simulink model "saturn_ib_stack_test"  (Simulink 6.2)
settings: Solver=ode4  SolverMode=SingleTasking  StartTime=-20.0  StopTime=620  FixedStep=0.005  RelTol=1e-3
values from neighbouring files (symbols this model uses):
  A_z_deg = 82.8200    (= 82.82)    [AS205_presettings.m]
  BN_1_sec = 14.4    [AS205_presettings.m]
  DeltaV_b_mps = 7.2381    [AS205_presettings.m]
  epsilon_2_sec = 15.0    (= 15)    [AS205_presettings.m]
  epsilon_prime_sec = 3.0    (= 3)    [AS205_presettings.m]
  i_deg = 28.89597    [AS205_presettings.m]
  lambda_0_deg = 102.32900    (= 102.329)    [AS205_presettings.m]
  lambda_L_deg = -80.561141    [AS205_presettings.m]
  pad_roll_L_deg = 100.0    (= 100)    [AS205_presettings.m]
  phi_L_deg = 28.521963    [AS205_presettings.m]
  phi_L_prime_deg = 28.360795    [AS205_presettings.m]
  R_L_m = 6373385.0    (= 6373385)    [AS205_presettings.m]
  R_T_m = 6570774.0    (= 6570774)    [AS205_presettings.m]
  T3_FM_sec = 6.08    [AS205_presettings.m]
  T_HSL_sec = 5.0    (= 5)    [AS205_presettings.m]
  Theta_T_deg = 0.000    (= 0)    [AS205_presettings.m]
  V_T_mps = 7780.976    [AS205_presettings.m]
  Xdotdot_VGT_mps2 = -9.251    [AS205_presettings.m]
undefined symbols (not defined in the file or in its folder): e0_0, e1_0, e2_0, e3_0, m, s
libraries: simulink x99, aerolibconvert x83, aerolibutil x63, aerolibtransform2 x34, aerolibasang x2, aerolibatmos2 x2, aerolib6dofsys x2
(part 4 of 7)

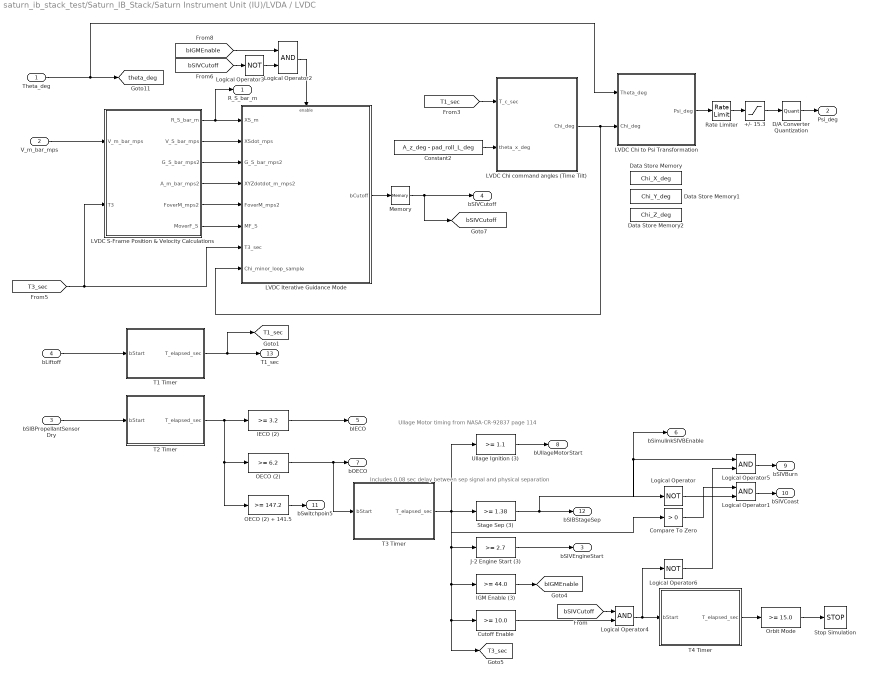
== system saturn_ib_stack_test/Saturn_IB_Stack/Saturn Instrument Unit (IU)/LVDA / LVDC ==
  note: Includes 0.08 sec delay between sep signal
      | and physical separation
  note: Ullage Motor timing
      | from NASA-CR-92837 page 114
  Theta_deg : Inport  Port=1  LatchInput=off
  V_m_bar_mps : Inport  Port=2  LatchInput=off
  bSIBPropellantSensorDry : Inport  Port=3  LatchInput=off
  bLiftoff : Inport  Port=4  PortDimensions=1  DataType=boolean  LatchInput=off
  +/- 15.3 : Saturate  UpperLimit=15.3  LowerLimit=-15.3
  Compare To Zero : simulink/Logic and Bit Operations/Compare To Zero  relop=>  LogicOutDataTypeMode=uint8  ZeroCross=off
  Constant2 : Constant  Value=A_z_deg - pad_roll_L_deg
  Cutoff Enable : simulink/Logic and Bit Operations/Compare To Constant  relop=>=  const=10.0  LogicOutDataTypeMode=boolean  ZeroCross=off
  D/A Converter Quantization : Quantizer  QuantizationInterval=0.0575
  Data Store Memory : DataStoreMemory  DataStoreName=Chi_X_deg  InitialValue=A_z_deg - pad_roll_L_deg  DataType=double
  Data Store Memory1 : DataStoreMemory  DataStoreName=Chi_Y_deg  InitialValue=0  DataType=double
  Data Store Memory2 : DataStoreMemory  DataStoreName=Chi_Z_deg  InitialValue=0  DataType=double
  IECO (2) : simulink/Logic and Bit Operations/Compare To Constant  relop=>=  const=3.2  LogicOutDataTypeMode=boolean  ZeroCross=off
  IGM Enable (3) : simulink/Logic and Bit Operations/Compare To Constant  relop=>=  const=44.0  LogicOutDataTypeMode=boolean  ZeroCross=off
  J-2 Engine Start (3) : simulink/Logic and Bit Operations/Compare To Constant  relop=>=  const=2.7  LogicOutDataTypeMode=boolean  ZeroCross=off
  LVDC Chi command angles (Time Tilt) : Subsystem
  LVDC Chi to Psi Transformation : Subsystem
  LVDC Iterative Guidance Mode : Subsystem  mask{lambda_dot_deg_per_sec=0.0, AP_dcm=[-0.18749569 -0.98223810 -0.73231298; 0.98202016 -0.18761026 0.20946740; -0.21948577 -0.32640360 0.99975374], T10_sec=286.9, A0_sec=458.9, A1=-1.194, Tr1=1.8, Tr2=0.0, Tr3=0.0, T2_sec=0.0, delta_T_sec=1.6, tau_1_i_preset_sec=286.9, tau_3_i_preset_sec=116.0, tau_3_preset_sec=262.52, V_ex1_mps=4135.6997, V_ex3_mps=4192.6960, PC0_sec=60.0, tau_1_0_sec=528.0, C_0_sec=35.0, Mdot_1_kg_per_sec=243.687, Mdot_3_kg_per_sec=204.129}
      mask prompts: lambda_dot_deg_per_sec "lambda_dot (deg/sec)"; AP_dcm "AP"; T10_sec "T_10 (sec)"; A0_sec "A0 (sec)"; T2_sec "T2 (sec)"; tau_1_i_preset_sec "T_1_i  preset (sec)"; tau_3_i_preset_sec "T_3_i preset (sec)"; tau_3_preset_sec "tau_3 preset (sec)"; V_ex1_mps "V_ex1 (m/sec)"; V_ex3_mps "V_ex3 (m/sec)"; PC0_sec "PC0 (sec)"; tau_1_0_sec "T_1_0 (sec)"; C_0_sec "C_0 (sec)"; Mdot_1_kg_per_sec "Mdot_1 (kg/sec)"; Mdot_3_kg_per_sec "Mdot_3 (kg/sec)"
      settings: PermitHierarchicalResolution=ParametersOnly
  LVDC S-Frame Position & Velocity Calculations : Subsystem  mask{delta_T_sec=1.6}
      mask prompts: delta_T_sec "Major Loop Time Interval (sec)"
  Logical Operator : Logic  Operator=NOT  AllPortsSameDT=off  OutDataTypeMode=Boolean
  Logical Operator{1..2,4..5} (4 alike) : Logic  AllPortsSameDT=off  OutDataTypeMode=Boolean
  Logical Operator3 : Logic  Operator=NOT  AllPortsSameDT=off  OutDataTypeMode=Boolean
  Logical Operator6 : Logic  Operator=NOT  AllPortsSameDT=off  OutDataTypeMode=Boolean
  Memory : Memory  InheritSampleTime=on
  OECO (2) : simulink/Logic and Bit Operations/Compare To Constant  relop=>=  const=6.2  LogicOutDataTypeMode=boolean  ZeroCross=off
  OECO (2) + 141.5 : simulink/Logic and Bit Operations/Compare To Constant  relop=>=  const=147.2  LogicOutDataTypeMode=boolean  ZeroCross=off
  Orbit Mode : simulink/Logic and Bit Operations/Compare To Constant  relop=>=  const=15.0  LogicOutDataTypeMode=boolean  ZeroCross=off
  Rate Limiter : RateLimiter  RisingSlewLimit=12.0  FallingSlewLimit=-12.0  SampleTimeMode=inherited
  Stage Sep (3) : simulink/Logic and Bit Operations/Compare To Constant  relop=>=  const=1.38  LogicOutDataTypeMode=boolean  ZeroCross=off
  Stop Simulation : Stop
  T1 Timer : Subsystem
  T2 Timer : Subsystem
  T3 Timer : Subsystem
  T4 Timer : Subsystem
  Ullage Ignition (3) : simulink/Logic and Bit Operations/Compare To Constant  relop=>=  const=1.1  LogicOutDataTypeMode=boolean  ZeroCross=off
  R_S_bar_m : Outport
  Psi_deg : Outport  Port=2
  bSIVEngineStart : Outport  Port=3
  bSIVCutoff : Outport  Port=4
  bIECO : Outport  Port=5
  bSimulinkSIVBEnable : Outport  Port=6
  bOECO : Outport  Port=7
  bUllageMotorStart : Outport  Port=8
  bSIVBurn : Outport  Port=9
  bSIVCoast : Outport  Port=10
  bSwitchpoin5 : Outport  Port=11
  bSIBStageSep : Outport  Port=12
  T1_sec : Outport  Port=13
  tag scope: T1_sec=global, T3_sec=global, bIGMEnable=global, bSIVCutoff=global, theta_deg=global
  wires:
  Constant2/1 -> LVDC Chi command angles (Time Tilt)/2(theta_x_deg)
  +/- 15.3/1 -> D/A Converter Quantization/1
  LVDC Chi to Psi Transformation/1(Psi_deg) -> Rate Limiter/1
  Theta_deg/1 -> LVDC Chi to Psi Transformation/1(Theta_deg), [theta_deg]
  [T1_sec] -> LVDC Chi command angles (Time Tilt)/1(T_c_sec)
  T2 Timer/1(T_elapsed_sec) -> IECO (2)/1, OECO (2)/1, OECO (2) + 141.5/1
  OECO (2)/1 -> T3 Timer/1(bStart), bOECO/1
  T3 Timer/1(T_elapsed_sec) -> Stage Sep (3)/1, Ullage Ignition (3)/1, Compare To Zero/1, J-2 Engine Start (3)/1, IGM Enable (3)/1, [T3_sec], Cutoff Enable/1
  Stage Sep (3)/1 -> bSimulinkSIVBEnable/1, Logical Operator/1, Logical Operator5/1, bSIBStageSep/1
  bLiftoff/1 -> T1 Timer/1(bStart)
  T1 Timer/1(T_elapsed_sec) -> [T1_sec], T1_sec/1
  Logical Operator/1 -> Logical Operator1/2
  Compare To Zero/1 -> Logical Operator1/1
  LVDC S-Frame Position & Velocity Calculations/2(V_S_bar_mps) -> LVDC Iterative Guidance Mode/2(XSdot_mps)
  LVDC S-Frame Position & Velocity Calculations/1(R_S_bar_m) -> R_S_bar_m/1, LVDC Iterative Guidance Mode/1(XS_m)
  LVDC S-Frame Position & Velocity Calculations/3(G_S_bar_mps2) -> LVDC Iterative Guidance Mode/3(G_S_bar_mps2)
  IGM Enable (3)/1 -> [bIGMEnable]
  LVDC S-Frame Position & Velocity Calculations/5(FoverM_mps2) -> LVDC Iterative Guidance Mode/5(FoverM_mps2)
  LVDC S-Frame Position & Velocity Calculations/4(A_m_bar_mps2) -> LVDC Iterative Guidance Mode/4(XYZdotdot_m_mps2)
  LVDC Chi command angles (Time Tilt)/1(Chi_deg) -> LVDC Chi to Psi Transformation/2(Chi_deg), LVDC Iterative Guidance Mode/8(Chi_minor_loop_sample)
  [T3_sec] -> LVDC Iterative Guidance Mode/7(T3_sec), LVDC S-Frame Position & Velocity Calculations/2(T3)
  LVDC S-Frame Position & Velocity Calculations/6(MoverF_S) -> LVDC Iterative Guidance Mode/6(MF_S)
  Rate Limiter/1 -> +/- 15.3/1
  LVDC Iterative Guidance Mode/1(bCutoff) -> Memory/1
  Logical Operator3/1 -> Logical Operator2/2
  [bSIVCutoff] -> Logical Operator3/1
  [bIGMEnable] -> Logical Operator2/1
  Logical Operator2/1 -> LVDC Iterative Guidance Mode/Enable
  V_m_bar_mps/1 -> LVDC S-Frame Position & Velocity Calculations/1(V_m_bar_mps)
  D/A Converter Quantization/1 -> Psi_deg/1
  Memory/1 -> bSIVCutoff/1, [bSIVCutoff]
  IECO (2)/1 -> bIECO/1
  bSIBPropellantSensorDry/1 -> T2 Timer/1(bStart)
  Ullage Ignition (3)/1 -> bUllageMotorStart/1
  OECO (2) + 141.5/1 -> bSwitchpoin5/1
  Logical Operator1/1 -> bSIVCoast/1
  J-2 Engine Start (3)/1 -> bSIVEngineStart/1
  T4 Timer/1(T_elapsed_sec) -> Orbit Mode/1
  Orbit Mode/1 -> Stop Simulation/1
  [bSIVCutoff] -> Logical Operator4/1
  Logical Operator4/1 -> T4 Timer/1(bStart), Logical Operator6/1
  Cutoff Enable/1 -> Logical Operator4/2
  Logical Operator5/1 -> bSIVBurn/1
  Logical Operator6/1 -> Logical Operator5/2

== system saturn_ib_stack_test/Saturn_IB_Stack/Saturn Instrument Unit (IU)/ST-124M Stabilized Platform ==
  note: ECI orientation of the ST-124M
      | platform at Ground Reference
      | Release time
  note: ECI Orientation of the L/V
  q_ECI : Inport  Port=1  LatchInput=off
  ST124M DCM : Inport  Port=2  LatchInput=off
  A_b_mps2 : Inport  Port=3  PortDimensions=3  LatchInput=off
  +/- 45.0 deg : Saturate  UpperLimit=pi/4.0  LowerLimit=-pi/4.0
  Accelerometer Quantization : Quantizer  QuantizationInterval=0.05
  Angle Conversion8 : aerolibconvert/Angle Conversion  IU=rad  OU=deg
  Body to ECI : Product  Multiplication=Matrix(*)  RndMeth=Zero
  Demux5 : Demux  Outputs=3
  ECI to Platform : Product  Multiplication=Matrix(*)  RndMeth=Zero
  Fine Resolver Quantization : Quantizer  QuantizationInterval=0.00279
  Integrating Accelerometers : Integrator
  Math Function : Math  Operator=transpose  SaturateOnIntegerOverflow=on
  Math Function1 : Math  Operator=transpose  SaturateOnIntegerOverflow=on
  Math Function2 : Math  Operator=transpose  SaturateOnIntegerOverflow=on
  Memory : Memory  X0=[A_z_deg - pad_roll_L_deg 0.0 0.0]  InheritSampleTime=on
  Mux : Mux  Inputs=3
  Platform Gimbal Angles : Subsystem  AncestorBlock=aerolibtransform2/Direction Cosine Matrix to Euler Angles
      mask Type: DCM2Euler
      mask Description: Determine equivalent ST-124M Gimbal angles from the 3-by-3 direction cosine matrix (DCM). The input DCM transforms vectors from Body frame to S-Frame.  EDD Equation 2.3.3 was used to determine the correct Euler angle rotation sequence used in the ST-124M.
      mask Display: disp('DCM2Gimbal')
  Product9 : Product  Multiplication=Matrix(*)  RndMeth=Zero
  Quaternions to  Direction Cosine Matrix1 : aerolibtransform2/Quaternions to  Direction Cosine Matrix
  Gimbal Angles (deg) : Outport
  accumulated velocity (m/sec) : Outport  Port=2  DataType=double
  wires:
  q_ECI/1 -> Quaternions to  Direction Cosine Matrix1/1
  Product9/1 -> Math Function2/1
  ST124M DCM/1 -> Math Function/1, ECI to Platform/1
  Quaternions to  Direction Cosine Matrix1/1 -> Product9/1, Math Function1/1
  Math Function/1 -> Product9/2
  Platform Gimbal Angles/1(ST-124 Gimbal) -> Demux5/1
  Demux5/2 -> Mux/2
  Demux5/3 -> +/- 45.0 deg/1
  Mux/1 -> Angle Conversion8/1
  Angle Conversion8/1 -> Fine Resolver Quantization/1
  +/- 45.0 deg/1 -> Mux/3
  Demux5/1 -> Mux/1
  ECI to Platform/1 -> Integrating Accelerometers/1
  Accelerometer Quantization/1 -> accumulated velocity (m/sec)/1
  Math Function1/1 -> Body to ECI/1
  Body to ECI/1 -> ECI to Platform/2
  A_b_mps2/1 -> Body to ECI/2
  Integrating Accelerometers/1 -> Accelerometer Quantization/1
  Fine Resolver Quantization/1 -> Memory/1
  Memory/1 -> Gimbal Angles (deg)/1
  Math Function2/1 -> Platform Gimbal Angles/1(DCM)

== system saturn_ib_stack_test/Saturn_IB_Stack/Initial Conditions/L/V Inertial Orientation/E-Frame to s-Frame (MES matrix) ==
  note: u(1)  sin Az
      | u(2)  sin Phi_L
      | u(3)  sin Theta_E
      | u(4)  cos Az
      | u(5)  cos Phi_L
      | u(6)  cos Theta_E
  note: Eqn 2.3.10
  Az phi_L Theta_E : Inport  Port=1  LatchInput=off
  11 : Fcn  Expr=u(5)*u(6)
  12 : Fcn  Expr=u(5)*u(3)
  13 : Fcn  Expr=u(2)
  21 : Fcn  Expr=u(2)*u(1)*u(6)-u(4)*u(3)
  22 : Fcn  Expr=u(2)*u(1)*u(3)+u(4)*u(6)
  23 : Fcn  Expr=-u(5)*u(1)
  31 : Fcn  Expr=-u(2)*u(4)*u(6)-u(1)*u(3)
  32 : Fcn  Expr=-u(2)*u(4)*u(3)+u(1)*u(6)
  33 : Fcn  Expr=u(5)*u(4)
  Mux : Mux  Inputs=2
  Mux2 : Mux  Inputs=9
  Reshape 9x1->3x3 : simulink/Math Operations/Reshape  OutputDimensionality=Customize  OutputDimensions=[3,3]
  SinCos3 : aerolibutil/SinCos
  DCM : Outport  InitialOutput=0
  wires:
  33/1 -> Mux2/9
  22/1 -> Mux2/5
  11/1 -> Mux2/1
  Mux2/1 -> Reshape 9x1->3x3/1
  Reshape 9x1->3x3/1 -> DCM/1
  Mux/1 -> 22/1, 11/1, 21/1, 31/1, 12/1, 32/1, 13/1, 33/1, 23/1
  23/1 -> Mux2/8
  13/1 -> Mux2/7
  32/1 -> Mux2/6
  12/1 -> Mux2/4
  31/1 -> Mux2/3
  21/1 -> Mux2/2
  Az phi_L Theta_E/1 -> SinCos3/1
  SinCos3/1 -> Mux/1
  SinCos3/2 -> Mux/2

== system saturn_ib_stack_test/Saturn_IB_Stack/Initial Conditions/MES Transform/MES Transform ==
  A_z_deg : Inport  Port=1  LatchInput=off
  phi_L_deg : Inport  Port=2  LatchInput=off
  Theta_E_deg : Inport  Port=3  LatchInput=off
  Angle Conversion2 : aerolibconvert/Angle Conversion  IU=deg  OU=rad
  E-Frame to s-Frame (MES matrix) : Subsystem  AncestorBlock="aerolibtransform2/Euler Angles to  Direction Cosine Matrix"
      mask Type: Euler2DCM
      mask Description: Determine the 3-by-3 direction cosine matrix (DCM) transforming the E-frame to the S-Frame
      mask Display: disp('MES')
  Mux : Mux  Inputs=3
  DCM : Outport
  wires:
  phi_L_deg/1 -> Mux/2
  Theta_E_deg/1 -> Mux/3
  A_z_deg/1 -> Mux/1
  Mux/1 -> Angle Conversion2/1
  E-Frame to s-Frame (MES matrix)/1(DCM) -> DCM/1
  Angle Conversion2/1 -> E-Frame to s-Frame (MES matrix)/1(Az phi_L Theta_E)

== system saturn_ib_stack_test/Saturn_IB_Stack/MES Transform/MES Transform/E-Frame to s-Frame (MES matrix) ==
  note: u(1)  sin Az
      | u(2)  sin Phi_L
      | u(3)  sin Theta_E
      | u(4)  cos Az
      | u(5)  cos Phi_L
      | u(6)  cos Theta_E
  note: Eqn 2.3.10
  Az phi_L Theta_E : Inport  Port=1  LatchInput=off
  11 : Fcn  Expr=u(5)*u(6)
  12 : Fcn  Expr=u(5)*u(3)
  13 : Fcn  Expr=u(2)
  21 : Fcn  Expr=u(2)*u(1)*u(6)-u(4)*u(3)
  22 : Fcn  Expr=u(2)*u(1)*u(3)+u(4)*u(6)
  23 : Fcn  Expr=-u(5)*u(1)
  31 : Fcn  Expr=-u(2)*u(4)*u(6)-u(1)*u(3)
  32 : Fcn  Expr=-u(2)*u(4)*u(3)+u(1)*u(6)
  33 : Fcn  Expr=u(5)*u(4)
  Mux : Mux  Inputs=2
  Mux2 : Mux  Inputs=9
  Reshape 9x1->3x3 : simulink/Math Operations/Reshape  OutputDimensionality=Customize  OutputDimensions=[3,3]
  SinCos3 : aerolibutil/SinCos
  DCM : Outport  InitialOutput=0
  wires:
  33/1 -> Mux2/9
  22/1 -> Mux2/5
  11/1 -> Mux2/1
  Mux2/1 -> Reshape 9x1->3x3/1
  Reshape 9x1->3x3/1 -> DCM/1
  Mux/1 -> 22/1, 11/1, 21/1, 31/1, 12/1, 32/1, 13/1, 33/1, 23/1
  23/1 -> Mux2/8
  13/1 -> Mux2/7
  32/1 -> Mux2/6
  12/1 -> Mux2/4
  31/1 -> Mux2/3
  21/1 -> Mux2/2
  Az phi_L Theta_E/1 -> SinCos3/1
  SinCos3/1 -> Mux/1
  SinCos3/2 -> Mux/2

== system saturn_ib_stack_test/Saturn_IB_Stack/On Pad/Initial Conditions/L/V Inertial Orientation ==
  A_z_deg : Inport  Port=1  LatchInput=off
  phi_L_deg : Inport  Port=2  LatchInput=off
  Theta_E_deg : Inport  Port=3  LatchInput=off
  Angle Conversion2 : aerolibconvert/Angle Conversion  IU=deg  OU=rad
  E-Frame to s-Frame (MES matrix) : Subsystem  AncestorBlock="aerolibtransform2/Euler Angles to  Direction Cosine Matrix"
      mask Type: Euler2DCM
      mask Description: Determine the 3-by-3 direction cosine matrix (DCM) transforming the E-frame to the S-Frame
      mask Display: disp('MES')
  Mux : Mux  Inputs=3
  DCM : Outport
  wires:
  phi_L_deg/1 -> Mux/2
  Theta_E_deg/1 -> Mux/3
  A_z_deg/1 -> Mux/1
  Mux/1 -> Angle Conversion2/1
  E-Frame to s-Frame (MES matrix)/1(DCM) -> DCM/1
  Angle Conversion2/1 -> E-Frame to s-Frame (MES matrix)/1(Az phi_L Theta_E)

== system saturn_ib_stack_test/Saturn_IB_Stack/On Pad/Initial Conditions/LLA to ECF ==
  lat (rad) : Inport  Port=1  LatchInput=off
  lon (rad) : Inport  Port=2  LatchInput=off
  h (m) : Inport  Port=3  LatchInput=off
  Add : Sum  OutScaling=2^-10
  Add1 : Sum  OutScaling=2^-10
  Bias : Bias  Bias=1.0
  Divide : Product  Inputs=*/  OutScaling=2^-10
  Divide1 : Product  Inputs=*/  OutScaling=2^-10
  Math Function : Math  Operator=square  SaturateOnIntegerOverflow=on
  Math Function1 : Math  Operator=square  SaturateOnIntegerOverflow=on
  Math Function2 : Math  Operator=square  SaturateOnIntegerOverflow=on
  Math Function3 : Math  Operator=sqrt  SaturateOnIntegerOverflow=on
  Mux : Mux  Inputs=3
  Product : Product  RndMeth=Zero
  Product1 : Product  Inputs=3  RndMeth=Zero
  Product2 : Product  Inputs=3  RndMeth=Zero
  Product3 : Product  RndMeth=Zero
  Product4 : Product  RndMeth=Zero
  SinCos : aerolibutil/SinCos
  SinCos1 : aerolibutil/SinCos
  Unary Minus : simulink/Math Operations/Unary Minus  DoSatur=off
  WGS-84 ECC^2 : Constant  Value=0.006694380004260806515  OutDataTypeMode=double
  WGS-84 major : Constant  Value=6378137.0  OutDataTypeMode=double
  WGS-84 minor : Constant  Value=6356752.3142  OutDataTypeMode=double
  XYZ (m) : Outport
  wires:
  WGS-84 major/1 -> Divide/1, Math Function2/1
  SinCos/1 -> Math Function/1, Product4/2
  WGS-84 ECC^2/1 -> Product/1
  Math Function/1 -> Product/2
  Product/1 -> Unary Minus/1
  Divide/1 -> Add/1, Product3/2  "N"
  h (m)/1 -> Add1/2, Add/2
  lat (rad)/1 -> SinCos/1
  lon (rad)/1 -> SinCos1/1
  Add/1 -> Product1/1, Product2/1
  SinCos/2 -> Product2/2, Product1/2
  SinCos1/2 -> Product1/3
  SinCos1/1 -> Product2/3
  Product1/1 -> Mux/1
  Mux/1 -> XYZ (m)/1
  Product2/1 -> Mux/2
  Product4/1 -> Mux/3
  WGS-84 minor/1 -> Math Function1/1
  Divide1/1 -> Product3/1
  Product3/1 -> Add1/1
  Add1/1 -> Product4/1
  Bias/1 -> Math Function3/1
  Unary Minus/1 -> Bias/1
  Math Function3/1 -> Divide/2
  Math Function1/1 -> Divide1/1
  Math Function2/1 -> Divide1/2

== system saturn_ib_stack_test/Saturn_IB_Stack/On Pad/Initial Conditions/MES Transform ==
  theta_GMST_0_deg : Inport  Port=1  LatchInput=off
  Constant2 : Constant  Value=A_z_deg
  Constant8 : Constant  Value=phi_L_deg
  Constant9 : Constant  Value=lambda_L_deg
  MES Transform : Subsystem  TreatAsAtomicUnit=on  SystemSampleTime=0.8
  Sum2 : Sum  Inputs=|++
  DCM : Outport
  wires:
  Constant2/1 -> MES Transform/1(A_z_deg)
  Constant8/1 -> MES Transform/2(phi_L_deg)
  Constant9/1 -> Sum2/1
  Sum2/1 -> MES Transform/3(Theta_E_deg)
  theta_GMST_0_deg/1 -> Sum2/2
  MES Transform/1(DCM) -> DCM/1

== system saturn_ib_stack_test/Saturn_IB_Stack/S-IB Stage/Custom Variable Mass 6DoF (Quaternion)/Calculate DCM & Euler Angles ==
  p q r : Inport  Port=1  LatchInput=off
  Initial quaternion : Inport  Port=2  LatchInput=off
  Quaternions to  Direction Cosine Matrix : aerolibtransform2/Quaternions to  Direction Cosine Matrix
  Quaternions to Euler Angles : aerolibtransform2/Quaternions to Euler Angles
  q0 q1 q2 q3 : Integrator  InitialConditionSource=external  InitialCondition=[e0_0 e1_0 e2_0 e3_0]
  qdot : Subsystem
  DCM : Outport
  Euler : Outport  Port=2
  q : Outport  Port=3
  wires:
  Quaternions to Euler Angles/1 -> Euler/1
  Quaternions to  Direction Cosine Matrix/1 -> DCM/1
  p q r/1 -> qdot/1(p q r)
  Initial quaternion/1 -> q0 q1 q2 q3/2
  q0 q1 q2 q3/1 -> Quaternions to  Direction Cosine Matrix/1, Quaternions to Euler Angles/1, qdot/2(q0 q1 q2 q3), q/1
  qdot/1(qdot) -> q0 q1 q2 q3/1

== system saturn_ib_stack_test/Saturn_IB_Stack/S-IB Stage/Custom Variable Mass 6DoF (Quaternion)/Calculate omega_dot ==
  p q r : Inport  Port=1  LatchInput=off
  "I, I_dot" : Inport  Port=2  LatchInput=off
  Moments : Inport  Port=3  LatchInput=off
  I x w : Subsystem
  I x w1 : Subsystem
  Product2 : Product  Inputs=/*  Multiplication=Matrix(*)  SaturateOnIntegerOverflow=on
  Reshape : simulink/Math Operations/Reshape  OutputDimensionality=1-D array  OutputDimensions=[1,1]
  Selector : Selector  InputType=Matrix  Elements=[1 2 1]  Rows=1:3  Columns=-1  InputPortWidth=2
  Selector1 : Selector  InputType=Matrix  Elements=[1 2 1]  Rows=4:6  Columns=-1  InputPortWidth=2
  Selector2 : Selector  InputType=Matrix  Elements=[1 2 1]  Rows=1:3  Columns=-1  InputPortWidth=2
  Sum2 : Sum  Inputs=+--  SaturateOnIntegerOverflow=on
  wx(Iw) : aerolibutil/3x3 Cross Product
  pdot qdot rdot : Outport
  wires:
  I x w/1(I * w) -> wx(Iw)/2
  wx(Iw)/1 -> Sum2/3
  Selector1/1 -> I x w1/1(I_dot)
  I x w1/1(Id * w) -> Sum2/2
  Moments/1 -> Sum2/1
  Sum2/1 -> Product2/2
  Product2/1 -> Reshape/1
  p q r/1 -> I x w1/2(p q r), wx(Iw)/1, I x w/1(p q r)
  "I, I_dot"/1 -> Selector1/1, Selector2/1, Selector/1
  Selector2/1 -> Product2/1
  Selector/1 -> I x w/2(Inertia)
  Reshape/1 -> pdot qdot rdot/1

== system saturn_ib_stack_test/Saturn_IB_Stack/S-IB Stage/Custom Variable Mass 6DoF (Quaternion)/transform to Inertial axes  ==
  x y z : Inport  Port=1  LatchInput=off
  transform coefficients : Inport  Port=2  LatchInput=off
  Product : Product  Multiplication=Matrix(*)  SaturateOnIntegerOverflow=on  InputSameDT=on
  Ve : Outport
  wires:
  Product/1 -> Ve/1
  transform coefficients/1 -> Product/1
  x y z/1 -> Product/2

== system saturn_ib_stack_test/Saturn_IB_Stack/S-IB Stage/H-1 Engine Cluster/Engine 1 ==
  note: S-IB Actuator model taken from NASA-CR-92837
  T0_sec : Inport  Port=1  LatchInput=off
  Cg_m : Inport  Port=2  PortDimensions=3  LatchInput=off
  A_actuator_cmd_deg : Inport  Port=3  PortDimensions=1  LatchInput=off
  B_actuator_cmd_deg : Inport  Port=4  PortDimensions=1  LatchInput=off
  bEngineStart : Inport  Port=5  PortDimensions=1  DataType=boolean  LatchInput=off
  bEngineCutoff : Inport  Port=6  PortDimensions=1  DataType=boolean  LatchInput=off
  3x3 Cross Product : aerolibutil/3x3 Cross Product
  A Actuator : TransferFcn  Denominator=[0.00001942 0.0007963 0.05576 1]
  Add : Sum  Inputs=+-  OutScaling=2^-10
  Angle Conversion{,1..3} (4 alike) : aerolibconvert/Angle Conversion  IU=deg  OU=rad
  B Actuator : TransferFcn  Denominator=[0.00001942 0.0007963 0.05576 1]
  Constant1 : Constant  Value=0.0
  Constant2 : Constant  Value=0.0
  Engine Mount Point Rotation : Constant  Value=[mpr_deg 0.0 0.0]
  Engine Performace Scaling Factor : Gain  Gain=899475.0 / 859000.0
  Euler Angles to  Direction Cosine Matrix{,1..3} (4 alike) : aerolibtransform2/Euler Angles to  Direction Cosine Matrix
  Gimbal Limits : Saturate  UpperLimit=8.0  LowerLimit=-8.0
  Gimbal Limits1 : Saturate  UpperLimit=8.0  LowerLimit=-8.0
  Installation location (m) : Constant  Value=r_m  OutDataTypeMode=double
  Mux : Mux  Inputs=3
  Mux1 : Mux  Inputs=3
  Neutral Thrust Alignment : Constant  Value=[-45.0 0.0 0.0]
  Neutral tilt Euler angles (deg) : Constant  Value=[0.0 -6.0 0.0]
  Product{,1..3} (4 alike) : Product  Multiplication=Matrix(*)  RndMeth=Zero
  Product4 : Product  RndMeth=Zero
  Product5 : Product  RndMeth=Zero
  Terminator : Terminator
  Thrust Decay : Lookup  InputValues=[0.0 0.2 0.3 0.5]  OutputValues=[1.0 0.05 0.03 0.0]  LookUpMeth=Interpolation-Use End Values
  Thrust vs. Time : Lookup  InputValues=[0.0 20.0 40.0 60.0 80.0 100.0 120.0 140.0]  OutputValues=[859000.0 895819.0 923597.0 956249.0 984994.0 997243.0 993749.0 979176.0]
  Triggered Timer : Subsystem
  m_dot : Constant  Value=347.3009
  F_N : Outport
  M_Nm : Outport  Port=2
  mdot_kg_sec : Outport  Port=3
  wires:
  Angle Conversion/1 -> Euler Angles to  Direction Cosine Matrix/1
  Neutral tilt Euler angles (deg)/1 -> Angle Conversion/1
  Cg_m/1 -> Add/2
  Installation location (m)/1 -> Add/1
  Add/1 -> 3x3 Cross Product/1
  3x3 Cross Product/1 -> M_Nm/1
  Euler Angles to  Direction Cosine Matrix/1 -> Product/1
  Product4/1 -> mdot_kg_sec/1
  Engine Mount Point Rotation/1 -> Angle Conversion1/1
  Angle Conversion1/1 -> Euler Angles to  Direction Cosine Matrix1/1
  Euler Angles to  Direction Cosine Matrix1/1 -> Product1/1
  Product1/1 -> 3x3 Cross Product/2, F_N/1
  A_actuator_cmd_deg/1 -> Gimbal Limits1/1
  Product/1 -> Product2/2
  Neutral Thrust Alignment/1 -> Angle Conversion2/1
  Angle Conversion2/1 -> Euler Angles to  Direction Cosine Matrix2/1
  Euler Angles to  Direction Cosine Matrix2/1 -> Product2/1
  A Actuator/1 -> Mux/2
  B Actuator/1 -> Mux/3
  Constant1/1 -> Mux/1
  Mux/1 -> Angle Conversion3/1
  Angle Conversion3/1 -> Euler Angles to  Direction Cosine Matrix3/1
  Euler Angles to  Direction Cosine Matrix3/1 -> Product3/1
  Product2/1 -> Product3/2
  Product3/1 -> Product1/2
  Gimbal Limits/1 -> B Actuator/1
  Gimbal Limits1/1 -> A Actuator/1
  bEngineCutoff/1 -> Triggered Timer/1(bStart)
  Triggered Timer/1(T_elapsed_sec) -> Thrust Decay/1
  Thrust Decay/1 -> Product4/2, Product5/2
  m_dot/1 -> Product4/1
  Constant2/1 -> Mux1/3, Mux1/2
  Product5/1 -> Mux1/1
  Mux1/1 -> Product/2
  Thrust vs. Time/1 -> Engine Performace Scaling Factor/1
  T0_sec/1 -> Thrust vs. Time/1
  Engine Performace Scaling Factor/1 -> Product5/1
  B_actuator_cmd_deg/1 -> Gimbal Limits/1
  bEngineStart/1 -> Terminator/1

== system saturn_ib_stack_test/Saturn_IB_Stack/S-IB Stage/H-1 Engine Cluster/Engine 2 ==
  note: S-IB Actuator model taken from NASA-CR-92837
  T0_sec : Inport  Port=1  LatchInput=off
  Cg_m : Inport  Port=2  PortDimensions=3  LatchInput=off
  A_actuator_cmd_deg : Inport  Port=3  PortDimensions=1  LatchInput=off
  B_actuator_cmd_deg : Inport  Port=4  PortDimensions=1  LatchInput=off
  bEngineStart : Inport  Port=5  PortDimensions=1  DataType=boolean  LatchInput=off
  bEngineCutoff : Inport  Port=6  PortDimensions=1  DataType=boolean  LatchInput=off
  3x3 Cross Product : aerolibutil/3x3 Cross Product
  A Actuator : TransferFcn  Denominator=[0.00001942 0.0007963 0.05576 1]
  Add : Sum  Inputs=+-  OutScaling=2^-10
  Angle Conversion{,1..3} (4 alike) : aerolibconvert/Angle Conversion  IU=deg  OU=rad
  B Actuator : TransferFcn  Denominator=[0.00001942 0.0007963 0.05576 1]
  Constant1 : Constant  Value=0.0
  Constant2 : Constant  Value=0.0
  Engine Mount Point Rotation : Constant  Value=[mpr_deg 0.0 0.0]
  Engine Performace Scaling Factor : Gain  Gain=879102.0 / 859000.0
  Euler Angles to  Direction Cosine Matrix{,1..3} (4 alike) : aerolibtransform2/Euler Angles to  Direction Cosine Matrix
  Gimbal Limits : Saturate  UpperLimit=8.0  LowerLimit=-8.0
  Gimbal Limits1 : Saturate  UpperLimit=8.0  LowerLimit=-8.0
  Installation location (m) : Constant  Value=r_m  OutDataTypeMode=double
  Mux : Mux  Inputs=3
  Mux1 : Mux  Inputs=3
  Neutral Thrust Alignment : Constant  Value=[-45.0 0.0 0.0]
  Neutral tilt Euler angles (deg) : Constant  Value=[0.0 6.0 0.0]
  Product{,1..3} (4 alike) : Product  Multiplication=Matrix(*)  RndMeth=Zero
  Product4 : Product  RndMeth=Zero
  Product5 : Product  RndMeth=Zero
  Terminator : Terminator
  Thrust Decay : Lookup  InputValues=[0.0 0.2 0.3 0.5]  OutputValues=[1.0 0.05 0.03 0.0]  LookUpMeth=Interpolation-Use End Values
  Thrust vs. Time : Lookup  InputValues=[0.0 20.0 40.0 60.0 80.0 100.0 120.0 140.0]  OutputValues=[859000.0 895819.0 923597.0 956249.0 984994.0 997243.0 993749.0 979176.0]
  Triggered Timer : Subsystem
  m_dot : Constant  Value=347.3009
  F_N : Outport
  M_Nm : Outport  Port=2
  mdot_kg_sec : Outport  Port=3
  wires:
  Angle Conversion/1 -> Euler Angles to  Direction Cosine Matrix/1
  Neutral tilt Euler angles (deg)/1 -> Angle Conversion/1
  Cg_m/1 -> Add/2
  Installation location (m)/1 -> Add/1
  Add/1 -> 3x3 Cross Product/1
  3x3 Cross Product/1 -> M_Nm/1
  Euler Angles to  Direction Cosine Matrix/1 -> Product/1
  Engine Mount Point Rotation/1 -> Angle Conversion1/1
  Angle Conversion1/1 -> Euler Angles to  Direction Cosine Matrix1/1
  Euler Angles to  Direction Cosine Matrix1/1 -> Product1/1
  Product1/1 -> 3x3 Cross Product/2, F_N/1
  A_actuator_cmd_deg/1 -> Gimbal Limits1/1
  B_actuator_cmd_deg/1 -> Gimbal Limits/1
  Product/1 -> Product2/2
  Neutral Thrust Alignment/1 -> Angle Conversion2/1
  Angle Conversion2/1 -> Euler Angles to  Direction Cosine Matrix2/1
  Euler Angles to  Direction Cosine Matrix2/1 -> Product2/1
  A Actuator/1 -> Mux/2
  B Actuator/1 -> Mux/3
  Constant1/1 -> Mux/1
  Angle Conversion3/1 -> Euler Angles to  Direction Cosine Matrix3/1
  Euler Angles to  Direction Cosine Matrix3/1 -> Product3/1
  Product2/1 -> Product3/2
  Product3/1 -> Product1/2
  Mux/1 -> Angle Conversion3/1
  Product4/1 -> mdot_kg_sec/1
  bEngineCutoff/1 -> Triggered Timer/1(bStart)
  Triggered Timer/1(T_elapsed_sec) -> Thrust Decay/1
  Engine Performace Scaling Factor/1 -> Product5/1
  Thrust Decay/1 -> Product4/2, Product5/2
  m_dot/1 -> Product4/1
  Constant2/1 -> Mux1/3, Mux1/2
  Product5/1 -> Mux1/1
  Mux1/1 -> Product/2
  Gimbal Limits/1 -> B Actuator/1
  Gimbal Limits1/1 -> A Actuator/1
  Thrust vs. Time/1 -> Engine Performace Scaling Factor/1
  T0_sec/1 -> Thrust vs. Time/1
  bEngineStart/1 -> Terminator/1

== system saturn_ib_stack_test/Saturn_IB_Stack/S-IB Stage/H-1 Engine Cluster/Engine 3 ==
  note: S-IB Actuator model taken from NASA-CR-92837
  T0_sec : Inport  Port=1  LatchInput=off
  Cg_m : Inport  Port=2  PortDimensions=3  LatchInput=off
  A_actuator_cmd_deg : Inport  Port=3  PortDimensions=1  LatchInput=off
  B_actuator_cmd_deg : Inport  Port=4  PortDimensions=1  LatchInput=off
  bEngineStart : Inport  Port=5  PortDimensions=1  DataType=boolean  LatchInput=off
  bEngineCutoff : Inport  Port=6  PortDimensions=1  DataType=boolean  LatchInput=off
  3x3 Cross Product : aerolibutil/3x3 Cross Product
  A Actuator : TransferFcn  Denominator=[0.00001942 0.0007963 0.05576 1]
  Add : Sum  Inputs=+-  OutScaling=2^-10
  Angle Conversion{,1..3} (4 alike) : aerolibconvert/Angle Conversion  IU=deg  OU=rad
  B Actuator : TransferFcn  Denominator=[0.00001942 0.0007963 0.05576 1]
  Constant1 : Constant  Value=0.0
  Constant2 : Constant  Value=0.0
  Engine Mount Point Rotation : Constant  Value=[mpr_deg 0.0 0.0]
  Engine Performace Scaling Factor : Gain  Gain=889110.0 / 859000.0
  Euler Angles to  Direction Cosine Matrix{,1..3} (4 alike) : aerolibtransform2/Euler Angles to  Direction Cosine Matrix
  Gimbal Limits : Saturate  UpperLimit=8.0  LowerLimit=-8.0
  Gimbal Limits1 : Saturate  UpperLimit=8.0  LowerLimit=-8.0
  Installation location (m) : Constant  Value=r_m  OutDataTypeMode=double
  Mux : Mux  Inputs=3
  Mux1 : Mux  Inputs=3
  Neutral Thrust Alignment : Constant  Value=[-45.0 0.0 0.0]
  Neutral tilt Euler angles (deg) : Constant  Value=[0.0 -6.0 0.0]
  Product{,1..3} (4 alike) : Product  Multiplication=Matrix(*)  RndMeth=Zero
  Product4 : Product  RndMeth=Zero
  Product5 : Product  RndMeth=Zero
  Terminator : Terminator
  Thrust Decay : Lookup  InputValues=[0.0 0.2 0.3 0.5]  OutputValues=[1.0 0.05 0.03 0.0]  LookUpMeth=Interpolation-Use End Values
  Thrust vs. Time : Lookup  InputValues=[0.0 20.0 40.0 60.0 80.0 100.0 120.0 140.0]  OutputValues=[859000.0 895819.0 923597.0 956249.0 984994.0 997243.0 993749.0 979176.0]
  Triggered Timer : Subsystem
  m_dot : Constant  Value=347.3009
  F_N : Outport
  M_Nm : Outport  Port=2
  mdot_kg_sec : Outport  Port=3
  wires:
  Angle Conversion/1 -> Euler Angles to  Direction Cosine Matrix/1
  Neutral tilt Euler angles (deg)/1 -> Angle Conversion/1
  Cg_m/1 -> Add/2
  Installation location (m)/1 -> Add/1
  Add/1 -> 3x3 Cross Product/1
  3x3 Cross Product/1 -> M_Nm/1
  Euler Angles to  Direction Cosine Matrix/1 -> Product/1
  Engine Mount Point Rotation/1 -> Angle Conversion1/1
  Angle Conversion1/1 -> Euler Angles to  Direction Cosine Matrix1/1
  Euler Angles to  Direction Cosine Matrix1/1 -> Product1/1
  Product1/1 -> 3x3 Cross Product/2, F_N/1
  A_actuator_cmd_deg/1 -> Gimbal Limits1/1
  B_actuator_cmd_deg/1 -> Gimbal Limits/1
  Product/1 -> Product2/2
  Neutral Thrust Alignment/1 -> Angle Conversion2/1
  Angle Conversion2/1 -> Euler Angles to  Direction Cosine Matrix2/1
  Euler Angles to  Direction Cosine Matrix2/1 -> Product2/1
  A Actuator/1 -> Mux/2
  B Actuator/1 -> Mux/3
  Constant1/1 -> Mux/1
  Mux/1 -> Angle Conversion3/1
  Angle Conversion3/1 -> Euler Angles to  Direction Cosine Matrix3/1
  Euler Angles to  Direction Cosine Matrix3/1 -> Product3/1
  Product2/1 -> Product3/2
  Product3/1 -> Product1/2
  Product4/1 -> mdot_kg_sec/1
  bEngineCutoff/1 -> Triggered Timer/1(bStart)
  Triggered Timer/1(T_elapsed_sec) -> Thrust Decay/1
  Engine Performace Scaling Factor/1 -> Product5/1
  Thrust Decay/1 -> Product4/2, Product5/2
  m_dot/1 -> Product4/1
  Constant2/1 -> Mux1/3, Mux1/2
  Product5/1 -> Mux1/1
  Mux1/1 -> Product/2
  Gimbal Limits/1 -> B Actuator/1
  Gimbal Limits1/1 -> A Actuator/1
  Thrust vs. Time/1 -> Engine Performace Scaling Factor/1
  T0_sec/1 -> Thrust vs. Time/1
  bEngineStart/1 -> Terminator/1

== system saturn_ib_stack_test/Saturn_IB_Stack/S-IB Stage/H-1 Engine Cluster/Engine 4 ==
  note: S-IB Actuator model taken from NASA-CR-92837
  T0_sec : Inport  Port=1  LatchInput=off
  Cg_m : Inport  Port=2  PortDimensions=3  LatchInput=off
  A_actuator_cmd_deg : Inport  Port=3  PortDimensions=1  LatchInput=off
  B_actuator_cmd_deg : Inport  Port=4  PortDimensions=1  LatchInput=off
  bEngineStart : Inport  Port=5  PortDimensions=1  DataType=boolean  LatchInput=off
  bEngineCutoff : Inport  Port=6  PortDimensions=1  DataType=boolean  LatchInput=off
  3x3 Cross Product : aerolibutil/3x3 Cross Product
  A Actuator : TransferFcn  Denominator=[0.00001942 0.0007963 0.05576 1]
  Add : Sum  Inputs=+-  OutScaling=2^-10
  Angle Conversion{,1..3} (4 alike) : aerolibconvert/Angle Conversion  IU=deg  OU=rad
  B Actuator : TransferFcn  Denominator=[0.00001942 0.0007963 0.05576 1]
  Constant1 : Constant  Value=0.0
  Constant2 : Constant  Value=0.0
  Engine Mount Point Rotation : Constant  Value=[mpr_deg 0.0 0.0]
  Engine Performace Scaling Factor : Gain  Gain=875099.0 / 859000.0
  Euler Angles to  Direction Cosine Matrix{,1..3} (4 alike) : aerolibtransform2/Euler Angles to  Direction Cosine Matrix
  Gimbal Limits : Saturate  UpperLimit=8.0  LowerLimit=-8.0
  Gimbal Limits1 : Saturate  UpperLimit=8.0  LowerLimit=-8.0
  Installation location (m) : Constant  Value=r_m  OutDataTypeMode=double
  Mux : Mux  Inputs=3
  Mux1 : Mux  Inputs=3
  Neutral Thrust Alignment : Constant  Value=[-45.0 0.0 0.0]
  Neutral tilt Euler angles (deg) : Constant  Value=[0.0 6.0 0.0]
  Product{,1..3} (4 alike) : Product  Multiplication=Matrix(*)  RndMeth=Zero
  Product4 : Product  RndMeth=Zero
  Product5 : Product  RndMeth=Zero
  Terminator : Terminator
  Thrust Decay : Lookup  InputValues=[0.0 0.2 0.3 0.5]  OutputValues=[1.0 0.05 0.03 0.0]  LookUpMeth=Interpolation-Use End Values
  Thrust vs. Time : Lookup  InputValues=[0.0 20.0 40.0 60.0 80.0 100.0 120.0 140.0]  OutputValues=[859000.0 895819.0 923597.0 956249.0 984994.0 997243.0 993749.0 979176.0]
  Triggered Timer : Subsystem
  m_dot : Constant  Value=347.3009
  F_N : Outport
  M_Nm : Outport  Port=2
  mdot_kg_sec : Outport  Port=3
  wires:
  Angle Conversion/1 -> Euler Angles to  Direction Cosine Matrix/1
  Neutral tilt Euler angles (deg)/1 -> Angle Conversion/1
  Cg_m/1 -> Add/2
  Installation location (m)/1 -> Add/1
  Add/1 -> 3x3 Cross Product/1
  3x3 Cross Product/1 -> M_Nm/1
  Euler Angles to  Direction Cosine Matrix/1 -> Product/1
  Engine Mount Point Rotation/1 -> Angle Conversion1/1
  Angle Conversion1/1 -> Euler Angles to  Direction Cosine Matrix1/1
  Euler Angles to  Direction Cosine Matrix1/1 -> Product1/1
  Product1/1 -> 3x3 Cross Product/2, F_N/1
  A_actuator_cmd_deg/1 -> Gimbal Limits1/1
  B_actuator_cmd_deg/1 -> Gimbal Limits/1
  Product/1 -> Product2/2
  Neutral Thrust Alignment/1 -> Angle Conversion2/1
  Angle Conversion2/1 -> Euler Angles to  Direction Cosine Matrix2/1
  Euler Angles to  Direction Cosine Matrix2/1 -> Product2/1
  A Actuator/1 -> Mux/2
  B Actuator/1 -> Mux/3
  Constant1/1 -> Mux/1
  Mux/1 -> Angle Conversion3/1
  Angle Conversion3/1 -> Euler Angles to  Direction Cosine Matrix3/1
  Euler Angles to  Direction Cosine Matrix3/1 -> Product3/1
  Product2/1 -> Product3/2
  Product3/1 -> Product1/2
  Product4/1 -> mdot_kg_sec/1
  bEngineCutoff/1 -> Triggered Timer/1(bStart)
  Triggered Timer/1(T_elapsed_sec) -> Thrust Decay/1
  Engine Performace Scaling Factor/1 -> Product5/1
  Thrust Decay/1 -> Product4/2, Product5/2
  m_dot/1 -> Product4/1
  Constant2/1 -> Mux1/3, Mux1/2
  Product5/1 -> Mux1/1
  Mux1/1 -> Product/2
  Gimbal Limits/1 -> B Actuator/1
  Gimbal Limits1/1 -> A Actuator/1
  Thrust vs. Time/1 -> Engine Performace Scaling Factor/1
  T0_sec/1 -> Thrust vs. Time/1
  bEngineStart/1 -> Terminator/1

== system saturn_ib_stack_test/Saturn_IB_Stack/S-IB Stage/H-1 Engine Cluster/Engine 5 ==
  T0_sec : Inport  Port=1  LatchInput=off
  Cg_m : Inport  Port=2  LatchInput=off
  bEngineStart : Inport  Port=3  PortDimensions=1  DataType=boolean  LatchInput=off
  bEngineCutoff : Inport  Port=4  PortDimensions=1  DataType=boolean  LatchInput=off
  3x3 Cross Product : aerolibutil/3x3 Cross Product
  Add : Sum  Inputs=+-  OutScaling=2^-10
  Angle Conversion : aerolibconvert/Angle Conversion  IU=deg  OU=rad
  Constant2 : Constant  Value=0.0
  Engine Performace Scaling Factor : Gain  Gain=880170.0 / 859000.0
  Euler Angles to  Direction Cosine Matrix : aerolibtransform2/Euler Angles to  Direction Cosine Matrix
  Installation location (m) : Constant  Value=[0.0 0.0 0.81]
  Mux : Mux  Inputs=3
  Neutral tilt Euler angles (deg) : Constant  Value=[0.0 -3.0 0.0]
  Product : Product  Multiplication=Matrix(*)  RndMeth=Zero
  Product1 : Product  RndMeth=Zero
  Product2 : Product  RndMeth=Zero
  Terminator : Terminator
  Thrust Decay : Lookup  InputValues=[0.0 0.2 0.3 0.5]  OutputValues=[1.0 0.05 0.03 0.0]  LookUpMeth=Interpolation-Use End Values
  Thrust vs. Time : Lookup  InputValues=[0.0 20.0 40.0 60.0 80.0 100.0 120.0 140.0]  OutputValues=[859000.0 895819.0 923597.0 956249.0 984994.0 997243.0 993749.0 979176.0]
  Triggered Timer : Subsystem
  m_dot : Constant  Value=347.3009
  Thrust_N : Outport
  Moment_Nm : Outport  Port=2
  mdot_kg_sec : Outport  Port=3
  wires:
  Angle Conversion/1 -> Euler Angles to  Direction Cosine Matrix/1
  Neutral tilt Euler angles (deg)/1 -> Angle Conversion/1
  Cg_m/1 -> Add/2
  Installation location (m)/1 -> Add/1
  3x3 Cross Product/1 -> Moment_Nm/1
  Euler Angles to  Direction Cosine Matrix/1 -> Product/1
  Product/1 -> Thrust_N/1, 3x3 Cross Product/2
  Add/1 -> 3x3 Cross Product/1
  Constant2/1 -> Mux/3, Mux/2
  bEngineCutoff/1 -> Triggered Timer/1(bStart)
  Triggered Timer/1(T_elapsed_sec) -> Thrust Decay/1
  Product1/1 -> Mux/1
  Thrust Decay/1 -> Product1/2, Product2/2
  m_dot/1 -> Product2/1
  Product2/1 -> mdot_kg_sec/1
  Mux/1 -> Product/2
  Thrust vs. Time/1 -> Engine Performace Scaling Factor/1
  T0_sec/1 -> Thrust vs. Time/1
  Engine Performace Scaling Factor/1 -> Product1/1
  bEngineStart/1 -> Terminator/1

== system saturn_ib_stack_test/Saturn_IB_Stack/S-IB Stage/H-1 Engine Cluster/Engine 6 ==
  T0_sec : Inport  Port=1  LatchInput=off
  Cg_m : Inport  Port=2  LatchInput=off
  bEngineStart : Inport  Port=3  PortDimensions=1  DataType=boolean  LatchInput=off
  bEngineCutoff : Inport  Port=4  PortDimensions=1  DataType=boolean  LatchInput=off
  3x3 Cross Product : aerolibutil/3x3 Cross Product
  Add : Sum  Inputs=+-  OutScaling=2^-10
  Angle Conversion : aerolibconvert/Angle Conversion  IU=deg  OU=rad
  Constant2 : Constant  Value=0.0
  Engine Performace Scaling Factor : Gain  Gain=889013.0 / 859000.0
  Euler Angles to  Direction Cosine Matrix : aerolibtransform2/Euler Angles to  Direction Cosine Matrix
  Installation location (m) : Constant  Value=[0.0 -0.81 0.0]
  Mux : Mux  Inputs=3
  Neutral tilt Eulker angles (deg) : Constant  Value=[0.0 0.0 -3.0]
  Product : Product  Multiplication=Matrix(*)  RndMeth=Zero
  Product1 : Product  RndMeth=Zero
  Product2 : Product  RndMeth=Zero
  Terminator : Terminator
  Thrust Decay : Lookup  InputValues=[0.0 0.2 0.3 0.5]  OutputValues=[1.0 0.05 0.03 0.0]  LookUpMeth=Interpolation-Use End Values
  Thrust vs. Time : Lookup  InputValues=[0.0 20.0 40.0 60.0 80.0 100.0 120.0 140.0]  OutputValues=[859000.0 895819.0 923597.0 956249.0 984994.0 997243.0 993749.0 979176.0]
  Triggered Timer : Subsystem
  m_dot : Constant  Value=347.3009
  Thrust_N : Outport
  Moment_Nm : Outport  Port=2
  mdot_kg_sec : Outport  Port=3
  wires:
  Angle Conversion/1 -> Euler Angles to  Direction Cosine Matrix/1
  Neutral tilt Eulker angles (deg)/1 -> Angle Conversion/1
  Cg_m/1 -> Add/2
  Installation location (m)/1 -> Add/1
  Add/1 -> 3x3 Cross Product/1
  3x3 Cross Product/1 -> Moment_Nm/1
  Euler Angles to  Direction Cosine Matrix/1 -> Product/1
  Product/1 -> 3x3 Cross Product/2, Thrust_N/1
  T0_sec/1 -> Thrust vs. Time/1
  Constant2/1 -> Mux/3, Mux/2
  bEngineCutoff/1 -> Triggered Timer/1(bStart)
  Triggered Timer/1(T_elapsed_sec) -> Thrust Decay/1
  Engine Performace Scaling Factor/1 -> Product1/1
  Product1/1 -> Mux/1
  Thrust Decay/1 -> Product1/2, Product2/2
  m_dot/1 -> Product2/1
  Product2/1 -> mdot_kg_sec/1
  Mux/1 -> Product/2
  Thrust vs. Time/1 -> Engine Performace Scaling Factor/1
  bEngineStart/1 -> Terminator/1

== system saturn_ib_stack_test/Saturn_IB_Stack/S-IB Stage/H-1 Engine Cluster/Engine 7 ==
  T0_sec : Inport  Port=1  LatchInput=off
  Cg_m : Inport  Port=2  LatchInput=off
  bEngineStart : Inport  Port=3  PortDimensions=1  DataType=boolean  LatchInput=off
  bEngineCutoff : Inport  Port=4  PortDimensions=1  DataType=boolean  LatchInput=off
  3x3 Cross Product : aerolibutil/3x3 Cross Product
  Add : Sum  Inputs=+-  OutScaling=2^-10
  Angle Conversion : aerolibconvert/Angle Conversion  IU=deg  OU=rad
  Constant2 : Constant  Value=0.0
  Engine Performace Scaling Factor : Gain  Gain=885241.0 / 859000.0
  Euler Angles to  Direction Cosine Matrix : aerolibtransform2/Euler Angles to  Direction Cosine Matrix
  Installation location (m) : Constant  Value=[0.0 0.0 -0.81]
  Mux : Mux  Inputs=3
  Neutral tilt Eulker angles (deg) : Constant  Value=[0.0 3.0 0.0]
  Product : Product  Multiplication=Matrix(*)  RndMeth=Zero
  Product1 : Product  RndMeth=Zero
  Product2 : Product  RndMeth=Zero
  Terminator : Terminator
  Thrust Decay : Lookup  InputValues=[0.0 0.2 0.3 0.5]  OutputValues=[1.0 0.05 0.03 0.0]  LookUpMeth=Interpolation-Use End Values
  Thrust vs. Time : Lookup  InputValues=[0.0 20.0 40.0 60.0 80.0 100.0 120.0 140.0]  OutputValues=[859000.0 895819.0 923597.0 956249.0 984994.0 997243.0 993749.0 979176.0]
  Triggered Timer : Subsystem
  m_dot : Constant  Value=347.3009
  Thrust_N : Outport
  Moment_Nm : Outport  Port=2
  mdot_kg_sec : Outport  Port=3
  wires:
  Angle Conversion/1 -> Euler Angles to  Direction Cosine Matrix/1
  Neutral tilt Eulker angles (deg)/1 -> Angle Conversion/1
  Cg_m/1 -> Add/2
  Installation location (m)/1 -> Add/1
  Add/1 -> 3x3 Cross Product/1
  3x3 Cross Product/1 -> Moment_Nm/1
  Euler Angles to  Direction Cosine Matrix/1 -> Product/1
  Product/1 -> 3x3 Cross Product/2, Thrust_N/1
  T0_sec/1 -> Thrust vs. Time/1
  Constant2/1 -> Mux/3, Mux/2
  Mux/1 -> Product/2
  bEngineCutoff/1 -> Triggered Timer/1(bStart)
  Triggered Timer/1(T_elapsed_sec) -> Thrust Decay/1
  Thrust vs. Time/1 -> Engine Performace Scaling Factor/1
  Product1/1 -> Mux/1
  Thrust Decay/1 -> Product1/2, Product2/2
  m_dot/1 -> Product2/1
  Product2/1 -> mdot_kg_sec/1
  Engine Performace Scaling Factor/1 -> Product1/1
  bEngineStart/1 -> Terminator/1

== system saturn_ib_stack_test/Saturn_IB_Stack/S-IB Stage/H-1 Engine Cluster/Engine 8 ==
  T0_sec : Inport  Port=1  LatchInput=off
  Cg_m : Inport  Port=2  LatchInput=off
  bEngineStart : Inport  Port=3  PortDimensions=1  DataType=boolean  LatchInput=off
  bEngineCutoff : Inport  Port=4  PortDimensions=1  DataType=boolean  LatchInput=off
  3x3 Cross Product : aerolibutil/3x3 Cross Product
  Add : Sum  Inputs=+-  OutScaling=2^-10
  Angle Conversion : aerolibconvert/Angle Conversion  IU=deg  OU=rad
  Constant2 : Constant  Value=0.0
  Engine Performace Scaling Factor : Gain  Gain=884484.0 / 859000.0
  Euler Angles to  Direction Cosine Matrix : aerolibtransform2/Euler Angles to  Direction Cosine Matrix
  Installation location (m) : Constant  Value=[0.0 0.81 0.0]
  Mux : Mux  Inputs=3
  Neutral tilt Eulker angles (deg) : Constant  Value=[0.0 0.0 3.0]
  Product : Product  Multiplication=Matrix(*)  RndMeth=Zero
  Product1 : Product  RndMeth=Zero
  Product2 : Product  RndMeth=Zero
  Terminator : Terminator
  Thrust Decay : Lookup  InputValues=[0.0 0.2 0.3 0.5]  OutputValues=[1.0 0.05 0.03 0.0]  LookUpMeth=Interpolation-Use End Values
  Thrust vs. Time : Lookup  InputValues=[0.0 20.0 40.0 60.0 80.0 100.0 120.0 140.0]  OutputValues=[859000.0 895819.0 923597.0 956249.0 984994.0 997243.0 993749.0 979176.0]
  Triggered Timer : Subsystem
  m_dot : Constant  Value=347.3009
  Thrust_N : Outport
  Moment_Nm : Outport  Port=2
  mdot_kg_sec : Outport  Port=3
  wires:
  Angle Conversion/1 -> Euler Angles to  Direction Cosine Matrix/1
  Neutral tilt Eulker angles (deg)/1 -> Angle Conversion/1
  Cg_m/1 -> Add/2
  Installation location (m)/1 -> Add/1
  Add/1 -> 3x3 Cross Product/1
  3x3 Cross Product/1 -> Moment_Nm/1
  Euler Angles to  Direction Cosine Matrix/1 -> Product/1
  Product/1 -> 3x3 Cross Product/2, Thrust_N/1
  T0_sec/1 -> Thrust vs. Time/1
  Constant2/1 -> Mux/3, Mux/2
  Mux/1 -> Product/2
  bEngineCutoff/1 -> Triggered Timer/1(bStart)
  Triggered Timer/1(T_elapsed_sec) -> Thrust Decay/1
  Thrust vs. Time/1 -> Engine Performace Scaling Factor/1
  Product1/1 -> Mux/1
  Thrust Decay/1 -> Product1/2, Product2/2
  m_dot/1 -> Product2/1
  Product2/1 -> mdot_kg_sec/1
  Engine Performace Scaling Factor/1 -> Product1/1
  bEngineStart/1 -> Terminator/1

== system saturn_ib_stack_test/Saturn_IB_Stack/S-IB Stage/Relative Wind/Incidence, Sideslip, & Airspeed ==
  Vb : Inport  Port=1  LatchInput=off
  Airspeed : Math  Operator=sqrt  SaturateOnIntegerOverflow=on
  Compare To Zero : simulink/Logic and Bit Operations/Compare To Zero  relop=>  LogicOutDataTypeMode=boolean  ZeroCross=off
  Constant : Constant  Value=0.0
  Demux : Demux  Outputs=2
  Dot Product : simulink/Math Operations/Dot Product  InputSameDT=on  OutDataType=sfix(16)  OutScaling=2^-10  DoSatur=off
  Incidence : Trigonometry  Operator=atan2
  Product : Product  Inputs=*/  SaturateOnIntegerOverflow=on
  Selector : Selector  Elements=2  InputPortWidth=3
  Selector1 : Selector  Elements=[3 1]  InputPortWidth=3
  Sideslip : Trigonometry  Operator=asin
  Switch : Switch  Criteria=u2 ~= 0
  Alpha : Outport  InitialOutput=0
  Beta : Outport  Port=2  InitialOutput=0
  V : Outport  Port=3  InitialOutput=0
  wires:
  Product/1 -> Sideslip/1
  Demux/1 -> Incidence/1
  Demux/2 -> Incidence/2
  Selector1/1 -> Demux/1
  Dot Product/1 -> Airspeed/1
  Airspeed/1 -> V/1, Product/2, Compare To Zero/1
  Incidence/1 -> Alpha/1
  Vb/1 -> Selector1/1, Dot Product/1, Dot Product/2, Selector/1
  Selector/1 -> Product/1
  Compare To Zero/1 -> Switch/2
  Sideslip/1 -> Switch/1
  Switch/1 -> Beta/1
  Constant/1 -> Switch/3

== system saturn_ib_stack_test/Saturn_IB_Stack/S-IB Stage/Retrorocket Motors/Time Since Engine Start ==
  bStart : Inport  Port=1  DataType=boolean  LatchInput=off
  Clock : Clock
      settings: Decimation=10
  Constant : Constant  Value=0.0
  Data Store Memory : DataStoreMemory  DataStoreName=A  InitialValue=-1  DataType=double
  Data Store Read : DataStoreRead  DataStoreName=A  SampleTime=0
  Sum : Sum  Inputs=|+-
  Switch : Switch  Threshold=0.0
  Timer Initialization : Subsystem  TreatAsAtomicUnit=on
  T_elapsed_sec : Outport
  wires:
  bStart/1 -> Timer Initialization/Trigger
  Clock/1 -> Timer Initialization/1(In1), Sum/1
  Switch/1 -> T_elapsed_sec/1
  Sum/1 -> Switch/1
  Data Store Read/1 -> Sum/2, Switch/2
  Constant/1 -> Switch/3

== system saturn_ib_stack_test/Saturn_IB_Stack/S-IVB Stage/APS I Module/APS Thruster II ==
  Fire : Inport  Port=1  LatchInput=off
  Cg_m : Inport  Port=2  PortDimensions=3  LatchInput=off
  3x3 Cross Product : aerolibutil/3x3 Cross Product
  Add : Sum  Inputs=+-  OutScaling=2^-10
  Constant2 : Constant  Value=[0.0 0.0 0.0]
  Installation location (m) : Constant  Value=r_m  OutDataTypeMode=double
  Switch : Switch  Criteria=u2 ~= 0
  Thruster Force : Constant  Value=F_N  OutDataTypeMode=double
  F_N : Outport
  M_Nm : Outport  Port=2
  wires:
  Cg_m/1 -> Add/2
  Installation location (m)/1 -> Add/1
  Add/1 -> 3x3 Cross Product/1
  3x3 Cross Product/1 -> M_Nm/1
  Switch/1 -> 3x3 Cross Product/2, F_N/1
  Thruster Force/1 -> Switch/1
  Constant2/1 -> Switch/3
  Fire/1 -> Switch/2

== system saturn_ib_stack_test/Saturn_IB_Stack/S-IVB Stage/APS I Module/APS Thruster IV ==
  Fire : Inport  Port=1  LatchInput=off
  Cg_m : Inport  Port=2  PortDimensions=3  LatchInput=off
  3x3 Cross Product : aerolibutil/3x3 Cross Product
  Add : Sum  Inputs=+-  OutScaling=2^-10
  Constant2 : Constant  Value=[0.0 0.0 0.0]
  Installation location (m) : Constant  Value=r_m  OutDataTypeMode=double
  Switch : Switch  Criteria=u2 ~= 0
  Thruster Force : Constant  Value=F_N  OutDataTypeMode=double
  F_N : Outport
  M_Nm : Outport  Port=2
  wires:
  Cg_m/1 -> Add/2
  Installation location (m)/1 -> Add/1
  Add/1 -> 3x3 Cross Product/1
  3x3 Cross Product/1 -> M_Nm/1
  Switch/1 -> 3x3 Cross Product/2, F_N/1
  Thruster Force/1 -> Switch/1
  Constant2/1 -> Switch/3
  Fire/1 -> Switch/2

== system saturn_ib_stack_test/Saturn_IB_Stack/S-IVB Stage/APS I Module/APS Thruster P ==
  Fire : Inport  Port=1  LatchInput=off
  Cg_m : Inport  Port=2  PortDimensions=3  LatchInput=off
  3x3 Cross Product : aerolibutil/3x3 Cross Product
  Add : Sum  Inputs=+-  OutScaling=2^-10
  Constant2 : Constant  Value=[0.0 0.0 0.0]
  Installation location (m) : Constant  Value=r_m  OutDataTypeMode=double
  Switch : Switch  Criteria=u2 ~= 0
  Thruster Force : Constant  Value=F_N  OutDataTypeMode=double
  F_N : Outport
  M_Nm : Outport  Port=2
  wires:
  Cg_m/1 -> Add/2
  Installation location (m)/1 -> Add/1
  Add/1 -> 3x3 Cross Product/1
  3x3 Cross Product/1 -> M_Nm/1
  Switch/1 -> 3x3 Cross Product/2, F_N/1
  Thruster Force/1 -> Switch/1
  Constant2/1 -> Switch/3
  Fire/1 -> Switch/2
